simulink model "dead reckon"  (R2023a)
settings: Solver=FixedStepDiscrete  StartTime=0.0  StopTime=10  FixedStep=0.01  RelTol=1e-3
model workspace (MAT data in the model file):
  ticksPerRot = 360
  wheelR = 0.052
libraries: mobileRoboticsTrainingLib x5
settings Model: Creator=khydf  LastModifiedBy=khydf

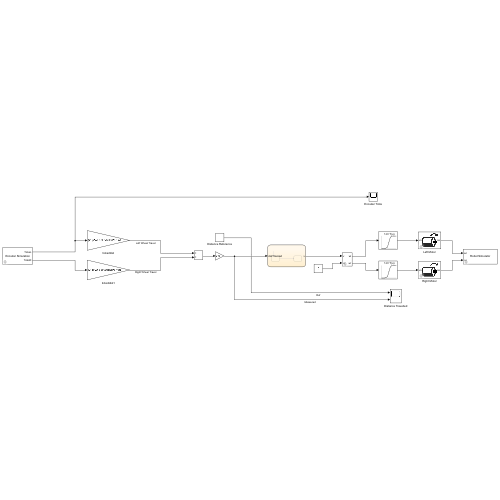
[thumbnail: Simulink's stored preview of the top-level diagram]
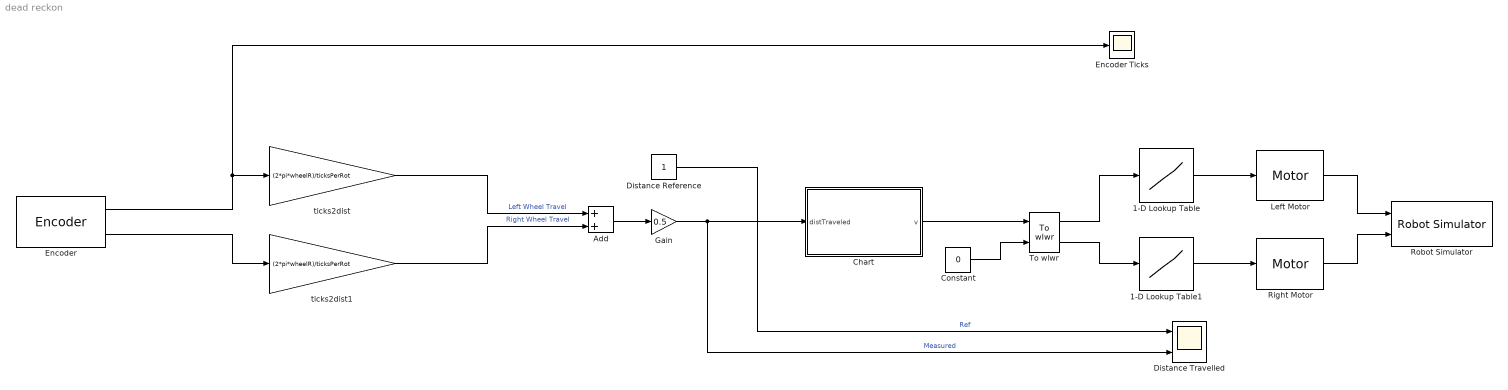
== system dead reckon ==
  1-D Lookup Table : Lookup_n-D  NumberOfTableDimensions=1  BreakpointsForDimension1=[-5:5]  Table=tanh([-5:5])  InternalRulePriority=Speed  RndMeth=Simplest
  1-D Lookup Table1 : Lookup_n-D  NumberOfTableDimensions=1  BreakpointsForDimension1=[-5:5]  Table=tanh([-5:5])  InternalRulePriority=Speed  RndMeth=Simplest
  Add : Sum
  Chart : Stateflow chart  TreatAsAtomicUnit=on
  Constant : Constant  Value=0
  Distance Reference : Constant
  Distance Travelled : Scope  NumInputPorts=2
  Encoder : mobileRoboticsTrainingLib/Encoder  axleLength=axleLength  wheelR=wheelR  ticksPerRot=ticksPerRot
      settings: SourceProductName=Mobile Robotics Training Library
  Encoder Ticks : Scope
  Gain : Gain  Gain=0.5
  Left Motor : mobileRoboticsTrainingLib/Motor  motorPlant=1  sensorType=Speed
      settings: SourceProductName=Mobile Robotics Training Library
  Right Motor : mobileRoboticsTrainingLib/Motor  motorPlant=1  sensorType=Speed
      settings: SourceProductName=Mobile Robotics Training Library
  Robot Simulator : mobileRoboticsTrainingLib/Robot Simulator  Priority=99  mapVar=[]  startX=0  startY=1  startTheta=0  axleLength=axleLength  wheelR=wheelR
  To wlwr : mobileRoboticsTrainingLib/To wlwr  axleLength=axleLength  wheelR=wheelR
  ticks2dist : Gain  Gain=(2*pi*wheelR)/ticksPerRot
  ticks2dist1 : Gain  Gain=(2*pi*wheelR)/ticksPerRot
  wires:
  Encoder/1 -> ticks2dist/1, Encoder Ticks/1
  ticks2dist/1 -> Add/1  "Left Wheel Travel"
  ticks2dist1/1 -> Add/2  "Right Wheel Travel"
  Encoder/2 -> ticks2dist1/1
  Add/1 -> Gain/1
  Gain/1 -> Distance Travelled/2, Chart/1(distTraveled)  "Measured"
  Chart/1(v) -> To wlwr/1
  Distance Reference/1 -> Distance Travelled/1  "Ref"
  Constant/1 -> To wlwr/2
  To wlwr/1 -> 1-D Lookup Table/1
  To wlwr/2 -> 1-D Lookup Table1/1
  1-D Lookup Table/1 -> Left Motor/1
  1-D Lookup Table1/1 -> Right Motor/1
  Left Motor/1 -> Robot Simulator/1
  Right Motor/1 -> Robot Simulator/2

== stateflow chart dead reckon/Chart ==
  state MoveForward
    v = 0.1
  state Stop
    v = 0
  (default) -> MoveForward : %Start
  MoveForward -> Stop : [distTraveled >= 1]
  data: distTraveled input; v output
